simulink model "ch6example8"  (Simulink 5.0)
settings: Solver=ode5  StartTime=0.0  StopTime=0.1  FixedStep=1/64000  RelTol=1e-3
libraries: dspbuff3 x2, commutil2 x2, commchan2 x1, dspsigattribs x1, simulink x1
settings Model: LastModifiedBy=shaoyubin

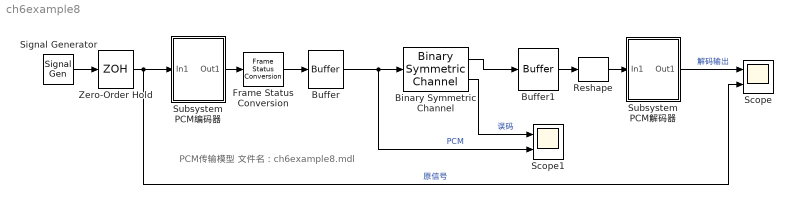
== system ch6example8 ==
  note: PCM传输模型
      | 文件名：ch6example8.mdl
  Binary Symmetric Channel : commchan2/Binary Symmetric Channel  P=0.01  s=71  E=on
  Buffer : dspbuff3/Buffer  N=1  V=0  ic=0
  Buffer1 : dspbuff3/Buffer  N=8  V=0  ic=0
  Frame Status Conversion : dspsigattribs/Frame Status Conversion  growRefPort=off  outframe=Frame-based
  Reshape : simulink/Math Operations/Reshape  OutputDimensionality=1-D array  OutputDimensions=[1,1]
  Scope : Scope  NumInputPorts=2
      settings: TimeRange=0.005  YMin=-1.1~-1.1  YMax=1.1~1.1
  Scope1 : Scope  NumInputPorts=2
      settings: TimeRange=0.005  YMin=-1~-5  YMax=2~5
  Signal Generator : SignalGenerator  Frequency=200
  Subsystem PCM编码器 : Subsystem
  Subsystem PCM解码器 : Subsystem
  Zero-Order Hold : ZeroOrderHold  SampleTime=1/8000
  wires:
  Signal Generator/1 -> Zero-Order Hold/1
  Subsystem PCM编码器/1(Out1) -> Frame Status Conversion/1
  Zero-Order Hold/1 -> Subsystem PCM编码器/1(In1), Scope/2  "原信号"
  Subsystem PCM解码器/1(Out1) -> Scope/1  "解码输出"
  Frame Status Conversion/1 -> Buffer/1
  Buffer1/1 -> Reshape/1
  Reshape/1 -> Subsystem PCM解码器/1(In1)
  Buffer/1 -> Binary Symmetric Channel/1, Scope1/2  "PCM"
  Binary Symmetric Channel/1 -> Buffer1/1
  Binary Symmetric Channel/2 -> Scope1/1  "误码"

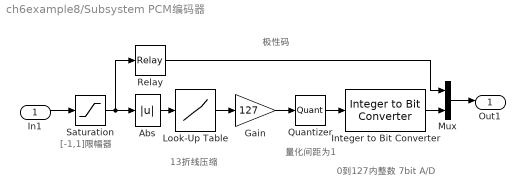
== system ch6example8/Subsystem PCM编码器 ==
  note: 0到127内整数
      | 7bit A/D
  note: [-1,1]限幅器
  note: 极性码
  note: 13折线压缩
  note: 量化间距为1
  In1 : Inport
  Abs : Abs  SaturateOnIntegerOverflow=on
  Gain : Gain  Gain=127  SaturateOnIntegerOverflow=on
  Integer to Bit Converter : commutil2/Integer to Bit Converter  nbits=7
  Look-Up Table : Lookup  InputValues=[-1,-1/2,-1/4,-1/8,-1/16,-1/32,-1/64,-1/128,0,1/128,1/64,1/32,1/16,1/8,1/4,1/2,1]  OutputValues=[-1:1/8:1]  SaturateOnIntegerOverflow=on
  Mux : Mux  Inputs=2
  Quantizer : Quantizer  QuantizationInterval=1
  Relay : Relay
  Saturation : Saturate  UpperLimit=1  LowerLimit=-1
  Out1 : Outport
  wires:
  Look-Up Table/1 -> Gain/1
  Quantizer/1 -> Integer to Bit Converter/1
  Gain/1 -> Quantizer/1
  Abs/1 -> Look-Up Table/1
  Relay/1 -> Mux/1
  Integer to Bit Converter/1 -> Mux/2
  Saturation/1 -> Abs/1, Relay/1
  Mux/1 -> Out1/1
  In1/1 -> Saturation/1

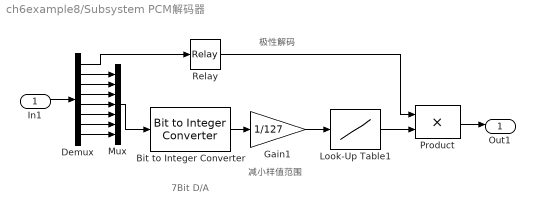
== system ch6example8/Subsystem PCM解码器 ==
  note: 极性解码
  note: 7Bit D/A
  note: 减小样值范围
  In1 : Inport
  Bit to Integer Converter : commutil2/Bit to Integer Converter  nbits=7
  Demux : Demux  Outputs=8
  Gain1 : Gain  Gain=1/127  SaturateOnIntegerOverflow=on
  Look-Up Table1 : Lookup  InputValues=[0:1/8:1]  OutputValues=[0,1/128,1/64,1/32,1/16,1/8,1/4,1/2,1]  SaturateOnIntegerOverflow=on
  Mux : Mux  Inputs=7
  Product : Product  SaturateOnIntegerOverflow=on
  Relay : Relay  OnSwitchValue=0.5  OffSwitchValue=0.5  OffOutputValue=-1
  Out1 : Outport
  wires:
  Bit to Integer Converter/1 -> Gain1/1
  Look-Up Table1/1 -> Product/2
  Relay/1 -> Product/1
  Mux/1 -> Bit to Integer Converter/1
  Demux/1 -> Relay/1
  Demux/2 -> Mux/1
  Demux/3 -> Mux/2
  Demux/8 -> Mux/7
  Demux/7 -> Mux/6
  Demux/6 -> Mux/5
  Demux/5 -> Mux/4
  Demux/4 -> Mux/3
  Gain1/1 -> Look-Up Table1/1
  In1/1 -> Demux/1
  Product/1 -> Out1/1
